simulink model "SimulacionKMotores"  (R2017b)
settings: Solver=VariableStepAuto  StartTime=0.0  StopTime=50000  RelTol=1e-3
undefined symbols (not defined in the file): A, B, C, K
settings Model: Creator=edgar  LastModifiedBy=edgar

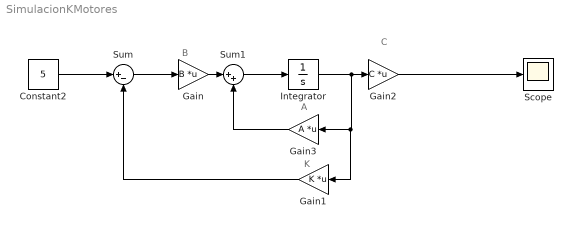
== system SimulacionKMotores ==
  note: K
  note: A
  note: C
  note: B
  Constant2 : Constant  Value=5
  Gain : Gain  Gain=B  Multiplication=Matrix(K*u)
  Gain1 : Gain  Gain=K  Multiplication=Matrix(K*u)
  Gain2 : Gain  Gain=C  Multiplication=Matrix(K*u)
  Gain3 : Gain  Gain=A  Multiplication=Matrix(K*u)
  Integrator : Integrator
  Scope : Scope
  Sum : Sum  Inputs=|+-
  Sum1 : Sum  Inputs=|++
  wires:
  Gain1/1 -> Sum/2
  Sum/1 -> Gain/1
  Constant2/1 -> Sum/1
  Gain/1 -> Sum1/1
  Gain3/1 -> Sum1/2
  Sum1/1 -> Integrator/1
  Integrator/1 -> Gain1/1, Gain3/1, Gain2/1
  Gain2/1 -> Scope/1
